simulink model "buck_boost_forceboost_withError"  (R2023b)
settings: Solver=VariableStepAuto  StartTime=0.0  StopTime=0.1  RelTol=1e-3
libraries: spsSeriesRLCBranchLib x5, spsMosfetLib x4, slpidlib x3, spsCurrentMeasurementLib x1, spsDCVoltageSourceLib x1, simulink x1, spsVoltageMeasurementLib x1, sps_lib x1
settings Model: Creator=sch  LastModifiedBy=sch

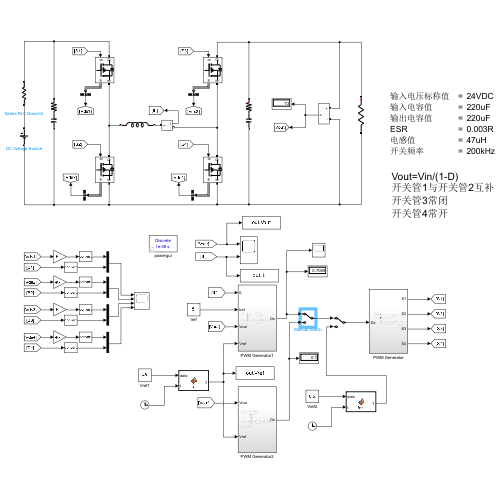
[thumbnail: Simulink's stored preview of the top-level diagram]
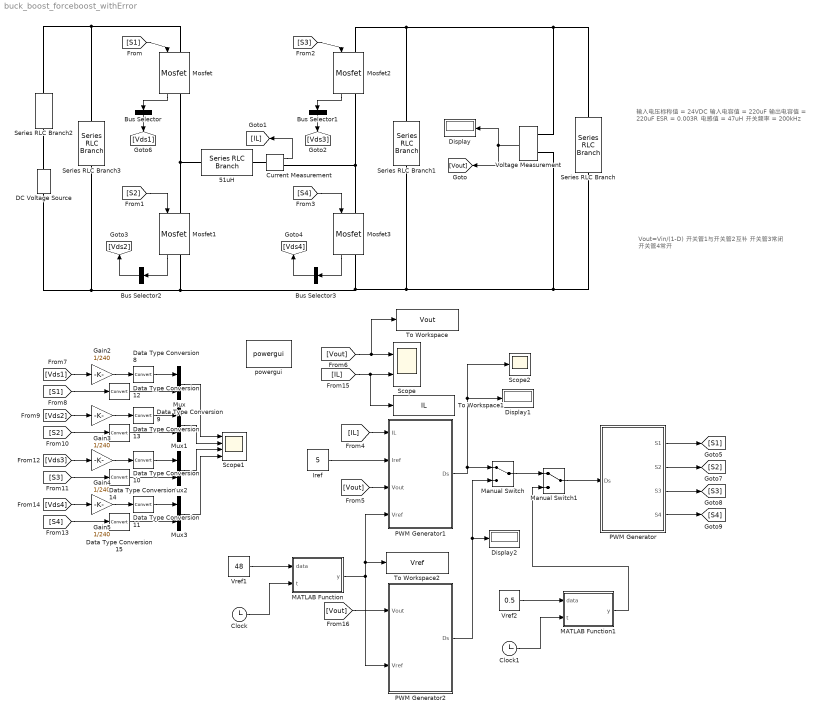
== system buck_boost_forceboost_withError ==
  note: Vout=Vin/(1-D)
      | 开关管1与开关管2互补
      | 开关管3常闭
      | 开关管4常开
  note: 输入电压标称值 = 24VDC
      | 输入电容值 = 220uF
      | 输出电容值 = 220uF
      | ESR = 0.003R
      | 电感值 = 47uH
      | 开关频率 = 200kHz
  51uH : spsSeriesRLCBranchLib/Series RLC Branch  LConnTagsString=__new0  RConnTagsString=__new0  BranchType=L  Resistance=1  Inductance=47e-6  SetiL0=on  InitialCurrent=2  Capacitance=1e-6  Setx0=off  InitialVoltage=0  Measurements=Branch current
  Bus Selector{,1..3} (4 alike) : BusSelector  OutputSignals=MOSFET voltage  OutputAsBus=on
  Clock : Clock
  Clock1 : Clock
  Current Measurement : spsCurrentMeasurementLib/Current Measurement  PhasorSimulation=off  OutputType=Complex  PSBequivalent=0
  DC Voltage Source : spsDCVoltageSourceLib/DC Voltage Source  Amplitude=24  Measurements=None
  Data Type Conversion{8..15} (8 alike) : DataTypeConversion  SaturateOnIntegerOverflow=off  RndMeth=Floor
  Display : Display
  Display1 : Display
  Display2 : Display
  Gain{2..5} (4 alike) : Gain  Gain=1/240
  Iref : Constant  Value=5
  MATLAB Function : MATLAB Function  TreatAsAtomicUnit=on
  MATLAB Function1 : MATLAB Function  TreatAsAtomicUnit=on
  Manual Switch : ManualSwitch
  Manual Switch1 : ManualSwitch
  Mosfet{,1..3} (4 alike) : spsMosfetLib/Mosfet  Ron=0.0063  Lon=0  Rd=0.001  Vfd=0  IC=0  Rs=1e5  Cs=inf  Measurements=on
  Mux{,1..3} (4 alike) : Mux  Inputs=2
  PWM Generator : Subsystem
  PWM Generator1 : Subsystem
  PWM Generator2 : Subsystem
  Scope : Scope  NumInputPorts=2
  Scope1 : Scope  NumInputPorts=4
  Scope2 : Scope
  Series RLC Branch : spsSeriesRLCBranchLib/Series RLC Branch  LConnTagsString=__new0  RConnTagsString=__new0  BranchType=R  Resistance=24  Inductance=1e-3  SetiL0=off  InitialCurrent=0  Capacitance=1e-6  Setx0=off  InitialVoltage=0  Measurements=None
  Series RLC Branch1 : spsSeriesRLCBranchLib/Series RLC Branch  LConnTagsString=__new0  RConnTagsString=__new0  BranchType=RC  Resistance=0.003  Inductance=5.6e-6  SetiL0=off  InitialCurrent=0  Capacitance=220e-6  Setx0=on  InitialVoltage=24  Measurements=None
  Series RLC Branch2 : spsSeriesRLCBranchLib/Series RLC Branch  LConnTagsString=__new0  RConnTagsString=__new0  BranchType=R  Resistance=1e-3  Inductance=1e-3  SetiL0=off  InitialCurrent=0  Capacitance=1e-6  Setx0=off  InitialVoltage=0  Measurements=None
  Series RLC Branch3 : spsSeriesRLCBranchLib/Series RLC Branch  LConnTagsString=__new0  RConnTagsString=__new0  BranchType=RC  Resistance=0.003  Inductance=5.6e-6  SetiL0=off  InitialCurrent=0  Capacitance=220e-6  Setx0=on  InitialVoltage=24  Measurements=None
  To Workspace : ToWorkspace  VariableName=Vout  SampleTime=-1
  To Workspace1 : ToWorkspace  VariableName=IL  SaveFormat=Timeseries  SampleTime=-1
  To Workspace2 : ToWorkspace  VariableName=Vref  SampleTime=-1
  Voltage Measurement : spsVoltageMeasurementLib/Voltage Measurement  PhasorSimulation=off  OutputType=Complex  PSBequivalent=0
  Vref1 : Constant  Value=48
  Vref2 : Constant  Value=0.5
  powergui : sps_lib/powergui  Priority=1  SimulationMode=Discrete  SampleTime=1e-8  frequency=60  Iterations=50  frequencyindice=0  Pbase=100e6  ErrMax=1e-4  UnitsV=kV  UnitsW=MW  buscounter=0  FunctionMessages=off  echomessages=off  EnableUseOfTLC=off  CurrentSourceSwitches=off  DisableSnubberDevices=off  DisableRonSwitches=off  DisableVfSwitches=off  DisplayEquations=off  AutomaticDiscreteSolvers=off  SolverType=Tustin/Backward Euler (TBE)  Interpol=off  ExternalGateDelay=off  methode=off  Ts=10  x0status=blocks  SPID=off  SwTol=0  HookPort=off  NonlinearTolerance=0  nMaxIteration=15  ContinueOnMaxIteration=off  RestoreLinks=warning  ResistiveCurrentMeasurement=off  Frange=[0:2:500]  Ylog=off  Xlog=on  ShowGrid=off  save=off  variable=ZData  structure=0  ZoomFFT=off  StartTime=0.0  cycles=1  DisplayStyle=1  fundamental=60  FreqAxis=off  MaxFrequency=1000  frequencyindicesteady=1  RmsSteady=1  display=off
  wires:
  Iref/1 -> PWM Generator1/2(Iref)
  Data Type Conversion13/1 -> Mux1/2
  Gain3/1 -> Data Type Conversion9/1
  [S3] -> Mosfet2/1
  Current Measurement/1 -> [IL]
  Data Type Conversion12/1 -> Mux/2
  PWM Generator/3(S3) -> [S3]
  [S2] -> Data Type Conversion13/1
  [S1] -> Mosfet/1
  [S4] -> Mosfet3/1
  Bus Selector1/1 -> [Vds3]
  PWM Generator/1(S1) -> [S1]
  Mosfet/1 -> Bus Selector/1
  Data Type Conversion15/1 -> Mux3/2
  Data Type Conversion8/1 -> Mux/1
  Bus Selector2/1 -> [Vds2]
  Data Type Conversion9/1 -> Mux1/1
  Voltage Measurement/1 -> [Vout], Display/1
  Mosfet2/1 -> Bus Selector1/1
  Data Type Conversion10/1 -> Mux2/1
  [Vds1] -> Gain2/1
  [S2] -> Mosfet1/1
  Bus Selector/1 -> [Vds1]
  Mosfet1/1 -> Bus Selector2/1
  Gain4/1 -> Data Type Conversion10/1
  Data Type Conversion14/1 -> Mux2/2
  [IL] -> To Workspace1/1, Scope/2
  Mux2/1 -> Scope1/3
  PWM Generator/4(S4) -> [S4]
  Gain2/1 -> Data Type Conversion8/1
  [Vds4] -> Gain5/1
  Data Type Conversion11/1 -> Mux3/1
  Bus Selector3/1 -> [Vds4]
  Mux/1 -> Scope1/1
  [S4] -> Data Type Conversion15/1
  PWM Generator/2(S2) -> [S2]
  Mosfet3/1 -> Bus Selector3/1
  [Vds3] -> Gain4/1
  [S3] -> Data Type Conversion14/1
  Mux3/1 -> Scope1/4
  [IL] -> PWM Generator1/1(IL)
  [Vout] -> PWM Generator1/3(Vout)
  [S1] -> Data Type Conversion12/1
  [Vds2] -> Gain3/1
  [Vout] -> To Workspace/1, Scope/1
  Mux1/1 -> Scope1/2
  PWM Generator1/1(Ds) -> Manual Switch/1, Display1/1, Scope2/1
  Gain5/1 -> Data Type Conversion11/1
  Vref1/1 -> MATLAB Function/1(data)
  Clock/1 -> MATLAB Function/2(t)
  MATLAB Function/1(y) -> PWM Generator2/2(Vref), To Workspace2/1, PWM Generator1/4(Vref)
  [Vout] -> PWM Generator2/1(Vout)
  Manual Switch/1 -> Manual Switch1/1
  Manual Switch1/1 -> PWM Generator/1(Ds)
  PWM Generator2/1(Ds) -> Display2/1, Manual Switch/2
  Clock1/1 -> MATLAB Function1/2(t)
  Vref2/1 -> MATLAB Function1/1(data)
  MATLAB Function1/1(y) -> Manual Switch1/2
  connections:
  Mosfet3/LConn1 -- Current Measurement/RConn1 -- Mosfet2/RConn1
  Series RLC Branch1/LConn1 -- Series RLC Branch/LConn1 -- Voltage Measurement/LConn1 -- Mosfet2/LConn1
  Mosfet1/LConn1 -- 51uH/LConn1 -- Mosfet/RConn1
  Series RLC Branch2/LConn1 -- Series RLC Branch3/LConn1 -- Mosfet/LConn1
  Series RLC Branch1/RConn1 -- Voltage Measurement/LConn2 -- Series RLC Branch/RConn1 -- DC Voltage Source/LConn1 -- Series RLC Branch3/RConn1 -- Mosfet1/RConn1 -- Mosfet3/RConn1
  51uH/RConn1 -- Current Measurement/LConn1
  DC Voltage Source/RConn1 -- Series RLC Branch2/RConn1

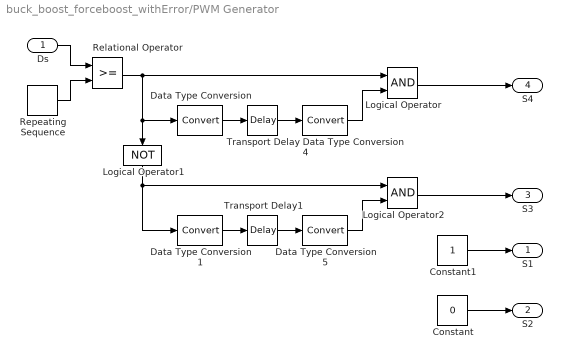
== system buck_boost_forceboost_withError/PWM Generator ==
  Ds : Inport
  Constant : Constant  Value=0
  Constant1 : Constant
  Data Type Conversion{,1,4..5} (4 alike) : DataTypeConversion  SaturateOnIntegerOverflow=off  RndMeth=Floor
  Logical Operator : Logic  AllPortsSameDT=off  OutDataTypeStr=boolean
  Logical Operator1 : Logic  Operator=NOT  AllPortsSameDT=off  OutDataTypeStr=boolean
  Logical Operator2 : Logic  AllPortsSameDT=off  OutDataTypeStr=boolean
  Relational Operator : RelationalOperator  OutDataTypeStr=boolean  InputSameDT=off
  Repeating Sequence : simulink/Sources/Repeating Sequence  rep_seq_t=[0 0.5/200000 1/200000]  rep_seq_y=[0 1 0]
  Transport Delay : TransportDelay  DelayTime=200e-9
  Transport Delay1 : TransportDelay  DelayTime=200e-9
  S1 : Outport
  S2 : Outport  Port=2
  S3 : Outport  Port=3
  S4 : Outport  Port=4
  wires:
  Ds/1 -> Relational Operator/1
  Repeating Sequence/1 -> Relational Operator/2
  Data Type Conversion/1 -> Transport Delay/1
  Data Type Conversion1/1 -> Transport Delay1/1
  Data Type Conversion5/1 -> Logical Operator2/2
  Data Type Conversion4/1 -> Logical Operator/2
  Relational Operator/1 -> Logical Operator/1, Data Type Conversion/1, Logical Operator1/1
  Logical Operator1/1 -> Data Type Conversion1/1, Logical Operator2/1
  Transport Delay1/1 -> Data Type Conversion5/1
  Transport Delay/1 -> Data Type Conversion4/1
  Constant1/1 -> S1/1
  Constant/1 -> S2/1
  Logical Operator2/1 -> S3/1
  Logical Operator/1 -> S4/1

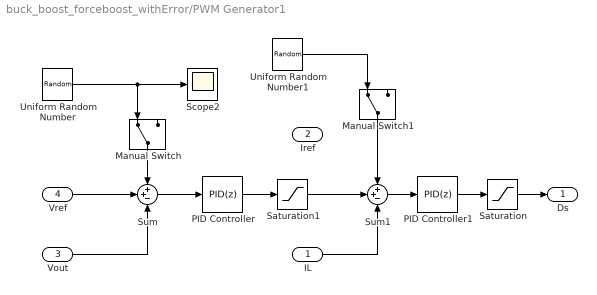
== system buck_boost_forceboost_withError/PWM Generator1 ==
  IL : Inport
  Iref : Inport  Port=2
  Vout : Inport  Port=3
  Vref : Inport  Port=4
  Manual Switch : ManualSwitch
  Manual Switch1 : ManualSwitch
  PID Controller : slpidlib/PID Controller  Controller=PID  Form=Parallel  TimeDomain=Discrete-time  UseExternalTs=off  SampleTime=1/200000  IntegratorMethod=Trapezoidal  FilterMethod=Forward Euler  ControllerParametersSource=internal  P=0.55  I=200  UseKiTs=off  D=0  N=100  UseFilter=on  TunerSelectOption=Transfer Function Based (PID Tuner App)  InitialConditionSource=internal  InitialConditionForIntegrator=0  InitialConditionForFilter=0  DifferentiatorICPrevScaledInput=0  ExternalReset=none  TrackingMode=off  Kt=1  LimitOutput=off  SatLimitsSource=internal  UpperSaturationLimit=inf  LowerSaturationLimit=-inf  LinearizeAsGain=on  AntiWindupMode=none  Kb=1  LimitIntegrator=off  UpperIntegratorSaturationLimit=inf  LowerIntegratorSaturationLimit=-inf  POutMin=[]  POutMax=[]  IOutMin=[]  IOutMax=[]  DOutMin=[]  DOutMax=[]  NOutMin=[]  NOutMax=[]  SumOutMin=[]  SumOutMax=[]  SaturationOutMin=[]  SaturationOutMax=[]  PParamMin=[]  PParamMax=[]  IParamMin=[]  IParamMax=[]  DParamMin=[]  DParamMax=[]  NParamMin=[]  NParamMax=[]  KbParamMin=[]  KbParamMax=[]  KtParamMin=[]  KtParamMax=[]  KbOutMin=[]  KbOutMax=[]  KtOutMin=[]  KtOutMax=[]  IntegratorOutMin=[]  IntegratorOutMax=[]  FilterOutMin=[]  FilterOutMax=[]  SumI1OutMin=[]  SumI1OutMax=[]  SumI2OutMin=[]  SumI2OutMax=[]  SumI3OutMin=[]  SumI3OutMax=[]  SumI4OutMin=[]  SumI4OutMax=[]  SumDOutMin=[]  SumDOutMax=[]  DifferentiatorOutMin=[]  DifferentiatorOutMax=[]  FilterDiffOutCoefMin=[]  FilterDiffOutCoefMax=[]  ReciprocalOutMin=[]  ReciprocalOutMax=[]  SumDenOutMin=[]  SumDenOutMax=[]  SumNumOutMin=[]  SumNumOutMax=[]  DivideOutMin=[]  DivideOutMax=[]  UdiffTsProdOutMin=[]  UdiffTsProdOutMax=[]  NTsProdOutMin=[]  NTsProdOutMax=[]  UintegralTsProdOutMin=[]  UintegralTsProdOutMax=[]  UngainTsProdOutMin=[]  UngainTsProdOutMax=[]  ClampingZeroOutDataTypeStr=Inherit: Inherit via back propagation  ClampingZeroOutMin=[]  ClampingZeroOutMax=[]  FilterDenConstantOutDataTypeStr=Inherit: Inherit via back propagation  FilterDenConstantOutMin=[]  FilterDenConstantOutMax=[]  PCopyOutDataTypeStr=Inherit: Inherit via back propagation  PCopyOutMin=[]  PCopyOutMax=[]  NCopyOutDataTypeStr=Inherit: Inherit via back propagation  NCopyOutMin=[]  NCopyOutMax=[]  IntegratorContinuousStateAttributes=''  IntegratorStateMustResolveToSignalObject=off  IntegratorRTWStateStorageClass=Auto  FilterContinuousStateAttributes=''  FilterStateMustResolveToSignalObject=off  FilterRTWStateStorageClass=Auto  ParallelPVariant=InternalParameters  IdealPVariant=Disabled  IVariant=InternalParameters  DVariant=InternalParameters  IntegratorVariant=Discrete  SatVariant=Disabled  AWVariant=Passthrough  PCopyVariant=Disabled  TRVariant=Disabled  FdbkBlocksVariant=Forward  IdealPFdbkVariant=Disabled  SatFdbkVariant=Disabled  DerivativeFilterVariant=ForwardEulerFilter  NVariant=InternalParameters  NCopyVariant=Disabled  FilterICVariant=InternalICsFilter  IntegratorICVariant=InternalICs  ExternalResetVariant=Disabled  TRSumVariant=Passthrough  SumFdbkVariant=Disabled  SumVariant=Sum_PID  TsampFilterVariant=InternalTs  TsampNgainVariant=Passthrough  TsampIntegralVariant=Disabled_SignalSpec  ExternalSaturationOutDataTypeStr=Inherit: Same as second input
  PID Controller1 : slpidlib/PID Controller  Controller=PID  Form=Parallel  TimeDomain=Discrete-time  UseExternalTs=off  SampleTime=1/200000  IntegratorMethod=Trapezoidal  FilterMethod=Forward Euler  ControllerParametersSource=internal  P=0.1  I=500  UseKiTs=off  D=0  N=100  UseFilter=off  TunerSelectOption=Transfer Function Based (PID Tuner App)  InitialConditionSource=internal  InitialConditionForIntegrator=0  InitialConditionForFilter=0  DifferentiatorICPrevScaledInput=0  ExternalReset=none  TrackingMode=off  Kt=1  LimitOutput=off  SatLimitsSource=internal  UpperSaturationLimit=inf  LowerSaturationLimit=-inf  LinearizeAsGain=on  AntiWindupMode=none  Kb=1  LimitIntegrator=off  UpperIntegratorSaturationLimit=inf  LowerIntegratorSaturationLimit=-inf  POutMin=[]  POutMax=[]  IOutMin=[]  IOutMax=[]  DOutMin=[]  DOutMax=[]  NOutMin=[]  NOutMax=[]  SumOutMin=[]  SumOutMax=[]  SaturationOutMin=[]  SaturationOutMax=[]  PParamMin=[]  PParamMax=[]  IParamMin=[]  IParamMax=[]  DParamMin=[]  DParamMax=[]  NParamMin=[]  NParamMax=[]  KbParamMin=[]  KbParamMax=[]  KtParamMin=[]  KtParamMax=[]  KbOutMin=[]  KbOutMax=[]  KtOutMin=[]  KtOutMax=[]  IntegratorOutMin=[]  IntegratorOutMax=[]  FilterOutMin=[]  FilterOutMax=[]  SumI1OutMin=[]  SumI1OutMax=[]  SumI2OutMin=[]  SumI2OutMax=[]  SumI3OutMin=[]  SumI3OutMax=[]  SumI4OutMin=[]  SumI4OutMax=[]  SumDOutMin=[]  SumDOutMax=[]  DifferentiatorOutMin=[]  DifferentiatorOutMax=[]  FilterDiffOutCoefMin=[]  FilterDiffOutCoefMax=[]  ReciprocalOutMin=[]  ReciprocalOutMax=[]  SumDenOutMin=[]  SumDenOutMax=[]  SumNumOutMin=[]  SumNumOutMax=[]  DivideOutMin=[]  DivideOutMax=[]  UdiffTsProdOutMin=[]  UdiffTsProdOutMax=[]  NTsProdOutMin=[]  NTsProdOutMax=[]  UintegralTsProdOutMin=[]  UintegralTsProdOutMax=[]  UngainTsProdOutMin=[]  UngainTsProdOutMax=[]  ClampingZeroOutDataTypeStr=Inherit: Inherit via back propagation  ClampingZeroOutMin=[]  ClampingZeroOutMax=[]  FilterDenConstantOutDataTypeStr=Inherit: Inherit via back propagation  FilterDenConstantOutMin=[]  FilterDenConstantOutMax=[]  PCopyOutDataTypeStr=Inherit: Inherit via back propagation  PCopyOutMin=[]  PCopyOutMax=[]  NCopyOutDataTypeStr=Inherit: Inherit via back propagation  NCopyOutMin=[]  NCopyOutMax=[]  IntegratorContinuousStateAttributes=''  IntegratorStateMustResolveToSignalObject=off  IntegratorRTWStateStorageClass=Auto  FilterContinuousStateAttributes=''  FilterStateMustResolveToSignalObject=off  FilterRTWStateStorageClass=Auto  ParallelPVariant=InternalParameters  IdealPVariant=Disabled  IVariant=InternalParameters  DVariant=InternalParameters  IntegratorVariant=Discrete  SatVariant=Disabled  AWVariant=Passthrough  PCopyVariant=Disabled  TRVariant=Disabled  FdbkBlocksVariant=Forward  IdealPFdbkVariant=Disabled  SatFdbkVariant=Disabled  DerivativeFilterVariant=Differentiator  NVariant=Passthrough  NCopyVariant=Disabled_SignalSpec  FilterICVariant=InternalICsDifferentiator  IntegratorICVariant=InternalICs  ExternalResetVariant=Disabled  TRSumVariant=Passthrough  SumFdbkVariant=Disabled  SumVariant=Sum_PID  TsampFilterVariant=InternalTs  TsampNgainVariant=Passthrough  TsampIntegralVariant=Disabled_SignalSpec  ExternalSaturationOutDataTypeStr=Inherit: Same as second input
  Saturation : Saturate  UpperLimit=0.8  LowerLimit=0.1
  Saturation1 : Saturate  UpperLimit=20  LowerLimit=-20
  Scope2 : Scope
  Sum : Sum  Inputs=++-
  Sum1 : Sum  Inputs=++-
  Uniform Random Number : UniformRandomNumber  Minimum=-0.05  Maximum=0.05  Seed=5624568  SampleTime=1/200000
  Uniform Random Number1 : UniformRandomNumber  Minimum=-0.05  Maximum=0.05  Seed=5624  SampleTime=1/200000
  Ds : Outport
  wires:
  Sum1/1 -> PID Controller1/1
  Saturation/1 -> Ds/1
  Sum/1 -> PID Controller/1
  PID Controller1/1 -> Saturation/1
  PID Controller/1 -> Saturation1/1
  Vout/1 -> Sum/3
  Vref/1 -> Sum/2
  Uniform Random Number/1 -> Manual Switch/1, Scope2/1
  Manual Switch/1 -> Sum/1
  Saturation1/1 -> Sum1/2
  IL/1 -> Sum1/3
  Uniform Random Number1/1 -> Manual Switch1/1
  Manual Switch1/1 -> Sum1/1

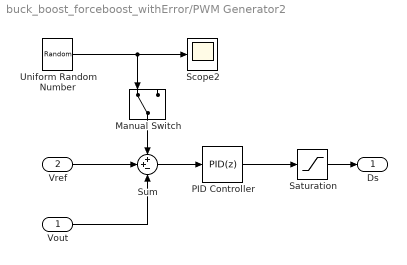
== system buck_boost_forceboost_withError/PWM Generator2 ==
  Vout : Inport
  Vref : Inport  Port=2
  Manual Switch : ManualSwitch
  PID Controller : slpidlib/PID Controller  Controller=PID  Form=Parallel  TimeDomain=Discrete-time  UseExternalTs=off  SampleTime=1/200000  IntegratorMethod=Trapezoidal  FilterMethod=Forward Euler  ControllerParametersSource=internal  P=0.01  I=1.5  UseKiTs=off  D=0  N=100  UseFilter=on  TunerSelectOption=Transfer Function Based (PID Tuner App)  InitialConditionSource=internal  InitialConditionForIntegrator=0  InitialConditionForFilter=0  DifferentiatorICPrevScaledInput=0  ExternalReset=none  TrackingMode=off  Kt=1  LimitOutput=off  SatLimitsSource=internal  UpperSaturationLimit=inf  LowerSaturationLimit=-inf  LinearizeAsGain=on  AntiWindupMode=none  Kb=1  LimitIntegrator=off  UpperIntegratorSaturationLimit=inf  LowerIntegratorSaturationLimit=-inf  POutMin=[]  POutMax=[]  IOutMin=[]  IOutMax=[]  DOutMin=[]  DOutMax=[]  NOutMin=[]  NOutMax=[]  SumOutMin=[]  SumOutMax=[]  SaturationOutMin=[]  SaturationOutMax=[]  PParamMin=[]  PParamMax=[]  IParamMin=[]  IParamMax=[]  DParamMin=[]  DParamMax=[]  NParamMin=[]  NParamMax=[]  KbParamMin=[]  KbParamMax=[]  KtParamMin=[]  KtParamMax=[]  KbOutMin=[]  KbOutMax=[]  KtOutMin=[]  KtOutMax=[]  IntegratorOutMin=[]  IntegratorOutMax=[]  FilterOutMin=[]  FilterOutMax=[]  SumI1OutMin=[]  SumI1OutMax=[]  SumI2OutMin=[]  SumI2OutMax=[]  SumI3OutMin=[]  SumI3OutMax=[]  SumI4OutMin=[]  SumI4OutMax=[]  SumDOutMin=[]  SumDOutMax=[]  DifferentiatorOutMin=[]  DifferentiatorOutMax=[]  FilterDiffOutCoefMin=[]  FilterDiffOutCoefMax=[]  ReciprocalOutMin=[]  ReciprocalOutMax=[]  SumDenOutMin=[]  SumDenOutMax=[]  SumNumOutMin=[]  SumNumOutMax=[]  DivideOutMin=[]  DivideOutMax=[]  UdiffTsProdOutMin=[]  UdiffTsProdOutMax=[]  NTsProdOutMin=[]  NTsProdOutMax=[]  UintegralTsProdOutMin=[]  UintegralTsProdOutMax=[]  UngainTsProdOutMin=[]  UngainTsProdOutMax=[]  ClampingZeroOutDataTypeStr=Inherit: Inherit via back propagation  ClampingZeroOutMin=[]  ClampingZeroOutMax=[]  FilterDenConstantOutDataTypeStr=Inherit: Inherit via back propagation  FilterDenConstantOutMin=[]  FilterDenConstantOutMax=[]  PCopyOutDataTypeStr=Inherit: Inherit via back propagation  PCopyOutMin=[]  PCopyOutMax=[]  NCopyOutDataTypeStr=Inherit: Inherit via back propagation  NCopyOutMin=[]  NCopyOutMax=[]  IntegratorContinuousStateAttributes=''  IntegratorStateMustResolveToSignalObject=off  IntegratorRTWStateStorageClass=Auto  FilterContinuousStateAttributes=''  FilterStateMustResolveToSignalObject=off  FilterRTWStateStorageClass=Auto  ParallelPVariant=InternalParameters  IdealPVariant=Disabled  IVariant=InternalParameters  DVariant=InternalParameters  IntegratorVariant=Discrete  SatVariant=Disabled  AWVariant=Passthrough  PCopyVariant=Disabled  TRVariant=Disabled  FdbkBlocksVariant=Forward  IdealPFdbkVariant=Disabled  SatFdbkVariant=Disabled  DerivativeFilterVariant=ForwardEulerFilter  NVariant=InternalParameters  NCopyVariant=Disabled  FilterICVariant=InternalICsFilter  IntegratorICVariant=InternalICs  ExternalResetVariant=Disabled  TRSumVariant=Passthrough  SumFdbkVariant=Disabled  SumVariant=Sum_PID  TsampFilterVariant=InternalTs  TsampNgainVariant=Passthrough  TsampIntegralVariant=Disabled_SignalSpec  ExternalSaturationOutDataTypeStr=Inherit: Same as second input
  Saturation : Saturate  UpperLimit=0.8  LowerLimit=0.1
  Scope2 : Scope
  Sum : Sum  Inputs=++-
  Uniform Random Number : UniformRandomNumber  Minimum=-0.05  Maximum=0.05  Seed=5624568  SampleTime=1/200000
  Ds : Outport
  wires:
  Saturation/1 -> Ds/1
  Sum/1 -> PID Controller/1
  PID Controller/1 -> Saturation/1
  Vout/1 -> Sum/3
  Vref/1 -> Sum/2
  Uniform Random Number/1 -> Manual Switch/1, Scope2/1
  Manual Switch/1 -> Sum/1

== matlab function buck_boost_forceboost_withError/MATLAB Function ==
  data: data input; t input; y output
function y = fcn(data, t)
if (t>=0)&(t<=0.04)
        y = data;
    elseif (t>0.04)&(t<=0.07)
        y = data*0.75;
    else
        y = data*1.5;
end

== matlab function buck_boost_forceboost_withError/MATLAB Function1 ==
  data: data input; t input; y output
function y = fcn(data, t)
if (t>=0)&(t<=0.04)
        y = data;
    elseif (t>0.04)&(t<=0.07)
        y = data*0.5;
    else
        y = data*1.33333;
end
